simulink model "beta_estimator_acceleration_driftingcar"  (R2017a)
settings: Solver=FixedStepAuto  StartTime=0.0  StopTime=10.0  FixedStep=0.01  RelTol=1e-3
undefined symbols (not defined in the file or in its folder): DiscIntNeverNeededParam
libraries: robotlib x5
settings Model: Creator=bascetta  LastModifiedBy=marco
settings OptimizationCC: PassReuseOutputArgsAs=Individual arguments  MaxStackSize=64
settings DebuggingCC: ParameterTunabilityLossMsg=error
settings HardwareCC: ProdBitPerPointer=32  ProdBitPerSizeT=32  ProdBitPerPtrDiffT=32  ProdLargestAtomicFloat=None  ProdIntDivRoundTo=Undefined  ProdEndianess=Unspecified  ProdWordSize=32  ProdHWDeviceType=Generic->Unspecified (assume 32-bit Generic)
settings SFSimCC: MATLABDynamicMemAlloc=off
settings RTWCC: SystemTargetFile=ert.tlc  HardwareBoard=Robot Operating System (ROS)  TLCOptions="-aInlineSetEventsForThisBaseRateFcn=TLC_FALSE -aSuppressMultiTaskScheduler=TLC_FALSE  -aRateBasedStepFcn=0"  TemplateMakefile=ert_default_tmf  Description=Embedded Coder  GenerateReport=on  Toolchain=Catkin  IncludeHyperlinkInReport=on  LaunchReport=on  TargetLang=C++  GenerateTraceInfo=on  GenerateTraceReport=on  GenerateTraceReportSl=on  GenerateTraceReportSf=on  GenerateTraceReportEml=on
settings CodeAppCC: ForceParamTrailComments=on  IgnoreCustomStorageClasses=off  OperatorAnnotations=on  SimulinkDataObjDesc=on  SFDataObjDesc=on  MATLABFcnDesc=on  InsertBlockDesc=on  MATLABSourceComments=on

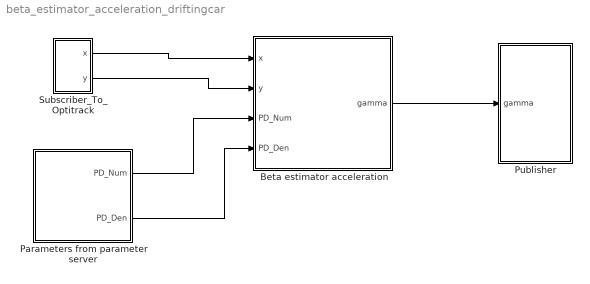
== system beta_estimator_acceleration_driftingcar ==
  Beta estimator acceleration : Subsystem
  Parameters from parameter server : Subsystem
  Publisher : Subsystem
  Subscriber_To_Optitrack : Subsystem
  wires:
  Beta estimator acceleration/1(gamma) -> Publisher/1(gamma)
  Subscriber_To_Optitrack/1(x) -> Beta estimator acceleration/1(x)
  Subscriber_To_Optitrack/2(y) -> Beta estimator acceleration/2(y)
  Parameters from parameter server/1(PD_Num) -> Beta estimator acceleration/3(PD_Num)
  Parameters from parameter server/2(PD_Den) -> Beta estimator acceleration/4(PD_Den)

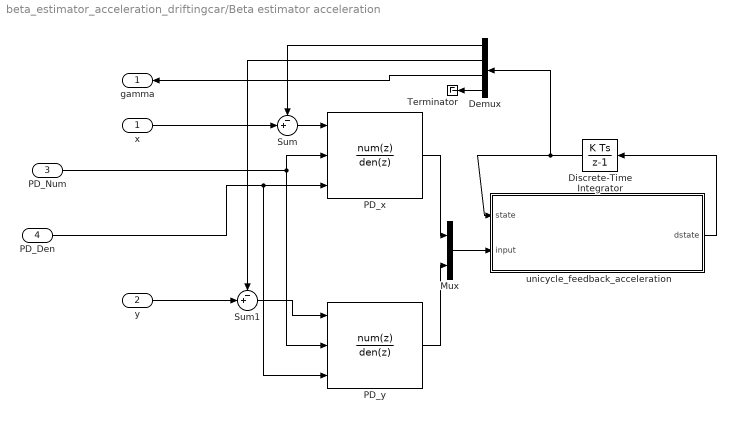
== system beta_estimator_acceleration_driftingcar/Beta estimator acceleration ==
  x : Inport
  y : Inport  Port=2
  PD_Num : Inport  Port=3
  PD_Den : Inport  Port=4
  Demux : Demux
  Discrete-Time Integrator : DiscreteIntegrator  InitialConditionSetting=State (most efficient)  SampleTime=-1  ICPrevOutput=DiscIntNeverNeededParam  ICPrevScaledInput=DiscIntNeverNeededParam
  Mux : Mux  Inputs=2
  PD_x : DiscreteTransferFcn  NumeratorSource=Input port  DenominatorSource=Input port  a0EqualsOne=on
      settings: InputPortMap=u0,p1,p3
  PD_y : DiscreteTransferFcn  NumeratorSource=Input port  DenominatorSource=Input port  a0EqualsOne=on
      settings: InputPortMap=u0,p1,p3
  Sum : Sum  Inputs=-+|
  Sum1 : Sum  Inputs=-+|
  Terminator : Terminator
  unicycle_feedback_acceleration : MATLAB Function  TreatAsAtomicUnit=on
  gamma : Outport
  wires:
  unicycle_feedback_acceleration/1(dstate) -> Discrete-Time Integrator/1
  Mux/1 -> unicycle_feedback_acceleration/2(input)
  Demux/1 -> Sum/1
  Sum1/1 -> PD_y/1
  Sum/1 -> PD_x/1
  PD_x/1 -> Mux/1
  y/1 -> Sum1/2
  Demux/3 -> gamma/1
  Demux/2 -> Sum1/1
  x/1 -> Sum/2
  PD_y/1 -> Mux/2
  Discrete-Time Integrator/1 -> Demux/1, unicycle_feedback_acceleration/1(state)
  Demux/4 -> Terminator/1
  PD_Num/1 -> PD_x/2, PD_y/2
  PD_Den/1 -> PD_y/3, PD_x/3

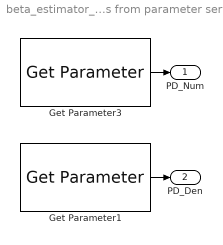
== system beta_estimator_acceleration_driftingcar/Parameters from parameter server ==
  Get Parameter1 : robotlib/Get Parameter  SourceLibraryInfo=This block requires Robotics System Toolbox  ParameterSource=Specify your own  ParameterName=/beta_estimator_acceleration_driftingcar/PD_Den  ParameterType=double  ParameterMaxArrayLength=16  ParameterInitialValue=0.0  SampleTime=-1  ShowErrorCodeOutput=off  ModelName=beta_estimator_acceleration_driftingcar  BlockId=ParamGet_beta_estimator_acceleration_driftingcar_74
      settings: SourceProductName=Robotics System Toolbox  SourceProductBaseCode=RO
  Get Parameter3 : robotlib/Get Parameter  SourceLibraryInfo=This block requires Robotics System Toolbox  ParameterSource=Specify your own  ParameterName=/beta_estimator_acceleration_driftingcar/PD_Num  ParameterType=double  ParameterMaxArrayLength=16  ParameterInitialValue=0.0  SampleTime=-1  ShowErrorCodeOutput=off  ModelName=beta_estimator_acceleration_driftingcar  BlockId=ParamGet_beta_estimator_acceleration_driftingcar_72
      settings: SourceProductName=Robotics System Toolbox  SourceProductBaseCode=RO
  PD_Num : Outport
  PD_Den : Outport  Port=2
  wires:
  Get Parameter3/1 -> PD_Num/1
  Get Parameter1/1 -> PD_Den/1

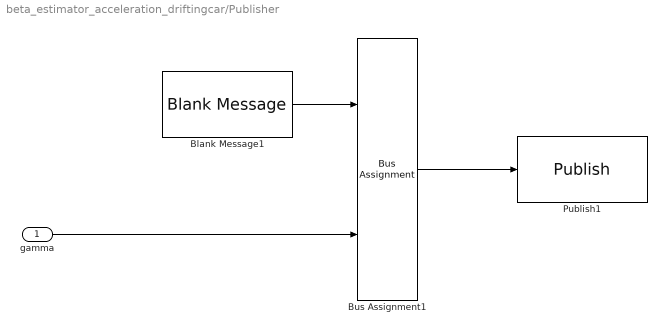
== system beta_estimator_acceleration_driftingcar/Publisher ==
  gamma : Inport
  Blank Message1 : robotlib/Blank Message  SourceLibraryInfo=This block requires Robotics System Toolbox  messageType=std_msgs/Float64  SampleTime=inf
      settings: SourceProductBaseCode=RO
  Bus Assignment1 : BusAssignment  AssignedSignals=Data
  Publish1 : robotlib/Publish  SourceLibraryInfo=This block requires Robotics System Toolbox  topicSource=Specify your own  topic=/gamma_estimator_acceleration  messageType=std_msgs/Float64  messageQueueLength=1
      settings: SourceProductBaseCode=RO
  wires:
  gamma/1 -> Bus Assignment1/2
  Blank Message1/1 -> Bus Assignment1/1
  Bus Assignment1/1 -> Publish1/1

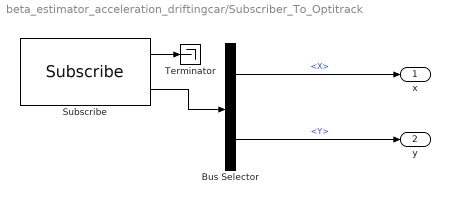
== system beta_estimator_acceleration_driftingcar/Subscriber_To_Optitrack ==
  Bus Selector : BusSelector  OutputSignals=X,Y
  Subscribe : robotlib/Subscribe  SourceLibraryInfo=This block requires Robotics System Toolbox  topicSource=Specify your own  topic=/car/ground_pose  messageType=geometry_msgs/Pose2D  sampleTime=-1  messageQueueLength=1
      settings: SourceProductBaseCode=RO
  Terminator : Terminator
  x : Outport
  y : Outport  Port=2
  wires:
  Subscribe/2 -> Bus Selector/1
  Subscribe/1 -> Terminator/1
  Bus Selector/1 -> x/1  "<X>"
  Bus Selector/2 -> y/1  "<Y>"

== matlab function beta_estimator_acceleration_driftingcar/Beta estimator acceleration/unicycle_feedback_acceleration ==
  data: state input size=4; dstate output size=4; input input size=2
function dstate = unicycle_feedback_acceleration(state,input)

% State and input variables
x     = state(1);
y     = state(2);
gamma = state(3); % theta+beta
v     = state(4);

ax    = input(1);
ay    = input(2);

% Model equations
dstate = zeros(4,1);
dstate(1) = v*cos(gamma);
dstate(2) = v*sin(gamma);
dstate(3) = (ay*cos(gamma)-ax*sin(gamma))/v;
dstate(4) = ax*cos(gamma)+ay*sin(gamma);
